simulink model "Controller"  (R2023a)
settings: Solver=VariableStepAuto  StartTime=0.0  StopTime=100  RelTol=1e-3
model workspace (MAT data in the model file):
  L = 1.5
  Tau = 3.5
  U = 0.1
values from neighbouring files (symbols this model uses):
  Kd = K(1)    [LQRSolver.m]
  Kgamma = K(3)    [LQRSolver.m]
  Ktheta = K(2)    [LQRSolver.m]
undefined symbols (not defined in the file or in its folder): pulse
libraries: simulink x1
settings Model: Creator=burnm  LastModifiedBy=burnm

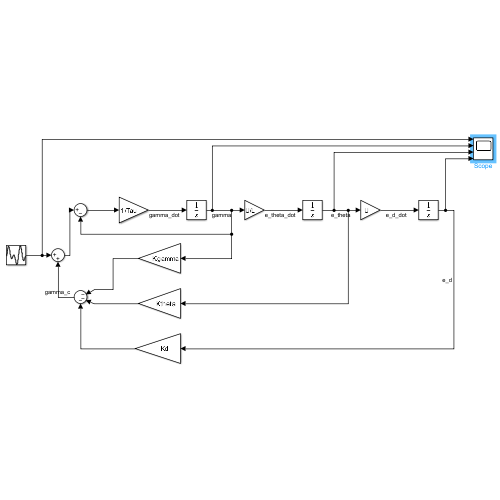
[thumbnail: Simulink's stored preview of the top-level diagram]
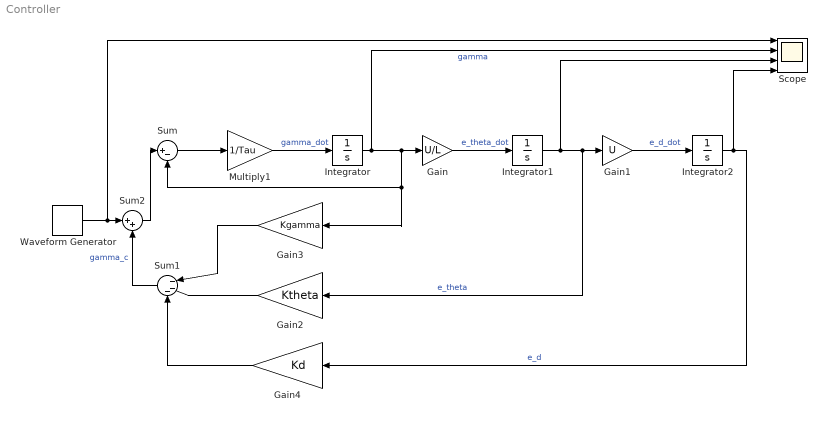
== system Controller ==
  Gain : Gain  Gain=U/L
  Gain1 : Gain  Gain=U
  Gain2 : Gain  Gain=Ktheta
  Gain3 : Gain  Gain=Kgamma
  Gain4 : Gain  Gain=Kd
  Integrator : Integrator
  Integrator1 : Integrator
  Integrator2 : Integrator
  Multiply1 : Gain  Gain=1/Tau
  Scope : Scope  NumInputPorts=4
  Sum : Sum  Inputs=|+-
  Sum1 : Sum  Inputs=|---
  Sum2 : Sum  Inputs=|++
  Waveform Generator : simulink/Sources/Waveform Generator  OutMin=[]  OutMax=[]  OutDataTypeStr=double  SelectedSignal=1  Signals=pulse(.1,0,20) + pulse(.1,40,20)  BlockNames=MultiportSwitch_1e6e4f2dc35a420  SampleTime=0.1
  wires:
  Multiply1/1 -> Integrator/1  "gamma_dot"
  Integrator/1 -> Scope/2, Sum/2, Gain3/1, Gain/1  "gamma"
  Gain/1 -> Integrator1/1  "e_theta_dot"
  Integrator1/1 -> Scope/3, Gain2/1, Gain1/1  "e_theta"
  Gain1/1 -> Integrator2/1  "e_d_dot"
  Integrator2/1 -> Scope/4, Gain4/1  "e_d"
  Gain2/1 -> Sum1/2
  Gain3/1 -> Sum1/1
  Gain4/1 -> Sum1/3
  Sum/1 -> Multiply1/1
  Waveform Generator/1 -> Scope/1, Sum2/1
  Sum1/1 -> Sum2/2  "gamma_c"
  Sum2/1 -> Sum/1
